simulink model "ControlSurf"  (R2016b)
settings: Solver=VariableStepAuto  StartTime=0.0  StopTime=10.0  RelTol=1e-3
libraries: Actuator_Lib x4
settings Model: ParameterArgumentNames=act  Creator=katiekwiz  LastModifiedBy=rega0051

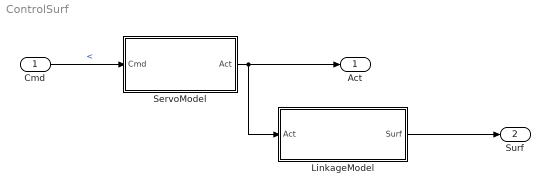
== system ControlSurf ==
  Cmd : Inport
  LinkageModel : Subsystem  Variant=on  VariantControl=Variant1  OverrideUsingVariant=VarLink_Pass
  ServoModel : Subsystem  Variant=on  VariantControl=Variant1  OverrideUsingVariant=VarServo_NL1
  Act : Outport
  Surf : Outport  Port=2
  wires:
  Cmd/1 -> ServoModel/1(Cmd)  "<"
  ServoModel/1(Act) -> LinkageModel/1("Act "), Act/1
  LinkageModel/1(" Surf") -> Surf/1

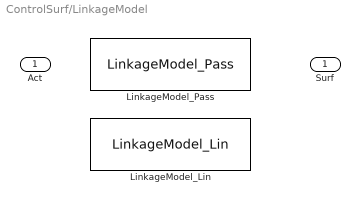
== system ControlSurf/LinkageModel ==
  "Act " : Inport
  LinkageModel_Lin : Actuator_Lib/LinkageModels/LinkageModel_Lin  VariantControl=VarLink_Lin  link=0
  LinkageModel_Pass : Actuator_Lib/LinkageModels/LinkageModel_Pass  VariantControl=VarLink_Pass
  " Surf" : Outport

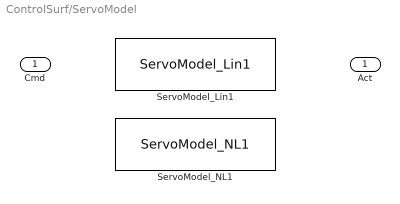
== system ControlSurf/ServoModel ==
  Cmd : Inport
  ServoModel_Lin1 : Actuator_Lib/ServoModels/ServoModel_Lin1  VariantControl=VarServo_Lin1  servo=servo
  ServoModel_NL1 : Actuator_Lib/ServoModels/ServoModel_NL1  VariantControl=VarServo_NL1  servo=servo
  Act : Outport
